simulink model "mylib2"  (R2018a)
settings: Solver=FixedStepAuto  StartTime=0.0  StopTime=10.0  RelTol=1e-3  SampleTimeConstraint=STIndependent
undefined symbols (not defined in the file or in its folder): In2, Mask_inport, Mask_outport, Out2
libraries: simulink x9
(part 2 of 2)

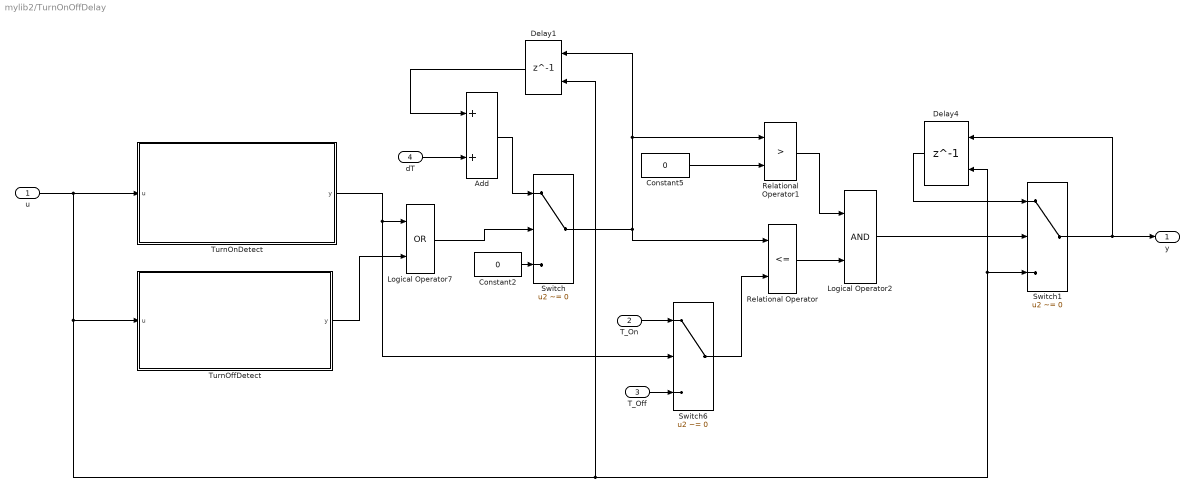
== system mylib2/TurnOnOffDelay ==
  u : Inport  OutDataTypeStr=boolean
  T_On : Inport  Port=2
  T_Off : Inport  Port=3
  dT : Inport  Port=4
  Add : Sum  RndMeth=Round  SaturateOnIntegerOverflow=on  InputSameDT=on  OutDataTypeStr=Inherit: Same as first input
  Constant2 : Constant  Value=0  OutDataTypeStr=Inherit: Inherit via back propagation
  Constant5 : Constant  Value=0  OutDataTypeStr=Inherit: Inherit via back propagation
  Delay1 : Delay  DelayLength=1  ExternalReset=Either
      settings: InputPortMap=u0,r5
  Delay4 : Delay  DelayLength=1  InitialConditionSource=Input port
      settings: InputPortMap=u0,p4
  Logical Operator2 : Logic  OutDataTypeStr=boolean
  Logical Operator7 : Logic  Operator=OR  OutDataTypeStr=boolean
  Relational Operator : RelationalOperator  Operator=<=  OutDataTypeStr=boolean  RndMeth=Simplest  InputSameDT=on
  Relational Operator1 : RelationalOperator  Operator=>  OutDataTypeStr=boolean  RndMeth=Simplest  InputSameDT=on
  Switch : Switch  Criteria=u2 ~= 0  RndMeth=Round  InputSameDT=on
  Switch1 : Switch  Criteria=u2 ~= 0
  Switch6 : Switch  Criteria=u2 ~= 0  RndMeth=Round  InputSameDT=on
  TurnOffDetect : Subsystem
  TurnOnDetect : Subsystem
  y : Outport  OutDataTypeStr=boolean
  wires:
  dT/1 -> Add/2
  Switch/1 -> Relational Operator1/1, Delay1/1, Relational Operator/1
  Delay1/1 -> Add/1
  Switch1/1 -> Delay4/1, y/1
  Add/1 -> Switch/1
  Logical Operator2/1 -> Switch1/2
  Constant2/1 -> Switch/3
  Relational Operator/1 -> Logical Operator2/2
  Relational Operator1/1 -> Logical Operator2/1
  Logical Operator7/1 -> Switch/2
  T_Off/1 -> Switch6/3
  T_On/1 -> Switch6/1
  Switch6/1 -> Relational Operator/2
  Constant5/1 -> Relational Operator1/2
  Delay4/1 -> Switch1/1
  u/1 -> Delay1/2, Delay4/2, Switch1/3, TurnOffDetect/1(u), TurnOnDetect/1(u)
  TurnOnDetect/1(y) -> Logical Operator7/1, Switch6/2
  TurnOffDetect/1(y) -> Logical Operator7/2

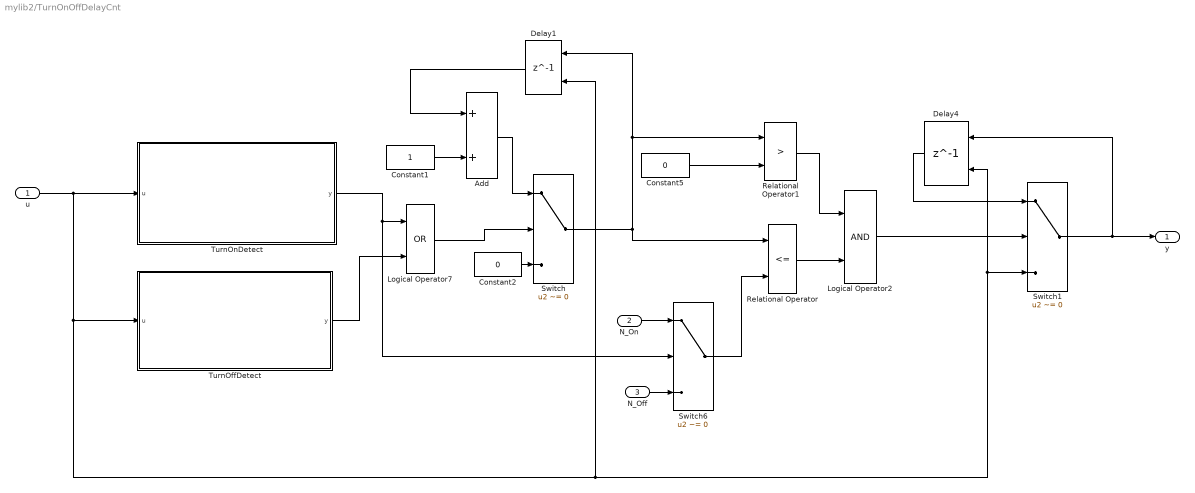
== system mylib2/TurnOnOffDelayCnt ==
  u : Inport  OutDataTypeStr=boolean
  N_On : Inport  Port=2
  N_Off : Inport  Port=3
  Add : Sum  RndMeth=Round  SaturateOnIntegerOverflow=on  InputSameDT=on  OutDataTypeStr=Inherit: Same as first input
  Constant1 : Constant  OutDataTypeStr=Inherit: Inherit via back propagation
  Constant2 : Constant  Value=0  OutDataTypeStr=Inherit: Inherit via back propagation
  Constant5 : Constant  Value=0  OutDataTypeStr=Inherit: Inherit via back propagation
  Delay1 : Delay  DelayLength=1  ExternalReset=Either
      settings: InputPortMap=u0,r5
  Delay4 : Delay  DelayLength=1  InitialConditionSource=Input port
      settings: InputPortMap=u0,p4
  Logical Operator2 : Logic  OutDataTypeStr=boolean
  Logical Operator7 : Logic  Operator=OR  OutDataTypeStr=boolean
  Relational Operator : RelationalOperator  Operator=<=  OutDataTypeStr=boolean  RndMeth=Simplest  InputSameDT=on
  Relational Operator1 : RelationalOperator  Operator=>  OutDataTypeStr=boolean  RndMeth=Simplest  InputSameDT=on
  Switch : Switch  Criteria=u2 ~= 0  RndMeth=Round  InputSameDT=on
  Switch1 : Switch  Criteria=u2 ~= 0
  Switch6 : Switch  Criteria=u2 ~= 0  RndMeth=Round  InputSameDT=on
  TurnOffDetect : Subsystem
  TurnOnDetect : Subsystem
  y : Outport  OutDataTypeStr=boolean
  wires:
  Constant1/1 -> Add/2
  Switch/1 -> Relational Operator1/1, Delay1/1, Relational Operator/1
  Delay1/1 -> Add/1
  Switch1/1 -> Delay4/1, y/1
  Add/1 -> Switch/1
  Logical Operator2/1 -> Switch1/2
  Constant2/1 -> Switch/3
  Relational Operator/1 -> Logical Operator2/2
  Relational Operator1/1 -> Logical Operator2/1
  Logical Operator7/1 -> Switch/2
  N_Off/1 -> Switch6/3
  N_On/1 -> Switch6/1
  Switch6/1 -> Relational Operator/2
  Constant5/1 -> Relational Operator1/2
  Delay4/1 -> Switch1/1
  u/1 -> Delay1/2, Delay4/2, Switch1/3, TurnOffDetect/1(u), TurnOnDetect/1(u)
  TurnOnDetect/1(y) -> Logical Operator7/1, Switch6/2
  TurnOffDetect/1(y) -> Logical Operator7/2

== system mylib2/twoAverage ==
  u1 : Inport
  u2 : Inport  Port=2
  Add : Sum  RndMeth=Round  SaturateOnIntegerOverflow=on  InputSameDT=on  OutDataTypeStr=Inherit: Same as first input
  Constant : Constant  Value=2  OutDataTypeStr=uint8
  Divide : Product  Inputs=*/  RndMeth=Round  SaturateOnIntegerOverflow=on  OutDataTypeStr=Inherit: Same as first input
  Divide1 : Product  Inputs=*/  RndMeth=Round  SaturateOnIntegerOverflow=on  OutDataTypeStr=Inherit: Same as first input
  y : Outport
  wires:
  Add/1 -> y/1
  u1/1 -> Divide/1
  Divide/1 -> Add/1
  Constant/1 -> Divide1/2, Divide/2
  u2/1 -> Divide1/1
  Divide1/1 -> Add/2

== system mylib2/F_M/Soft ==
  df : Inport  LibraryBlock=Mask_inport/In2  OutDataTypeStr=boolean
  frz : Inport  LibraryBlock=Mask_inport/In2  Port=2  OutDataTypeStr=boolean
  Delay : Delay  DelayLength=1  InitialConditionSource=Input port
      settings: InputPortMap=u0,p4
  Switch : Switch  Criteria=u2 ~= 0  InputSameDT=on
  F_M_xxx_fault_soft : Outport
  wires:
  frz/1 -> Switch/2
  Switch/1 -> Delay/1, F_M_xxx_fault_soft/1
  df/1 -> Delay/2, Switch/3
  Delay/1 -> Switch/1

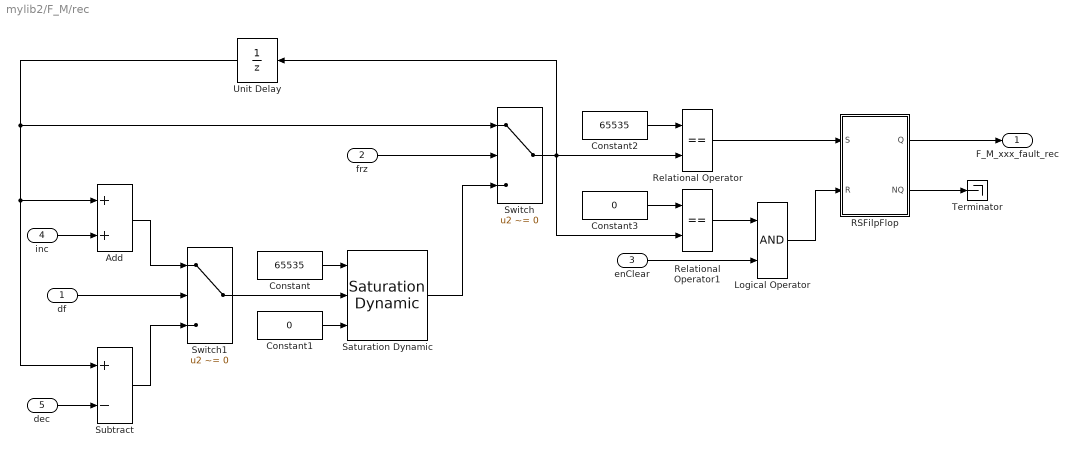
== system mylib2/F_M/rec ==
  df : Inport  LibraryBlock=Mask_inport/In2  OutDataTypeStr=boolean
  frz : Inport  LibraryBlock=Mask_inport/In2  Port=2  OutDataTypeStr=boolean
  enClear : Inport  LibraryBlock=Mask_inport/In2  Port=3  OutDataTypeStr=boolean
  inc : Inport  LibraryBlock=Mask_inport/In2  Port=4  OutDataTypeStr=uint16
  dec : Inport  LibraryBlock=Mask_inport/In2  Port=5  OutDataTypeStr=uint16
  Add : Sum  SaturateOnIntegerOverflow=on  InputSameDT=on  OutDataTypeStr=Inherit: Same as first input
  Constant : Constant  Value=65535  OutDataTypeStr=uint16
  Constant1 : Constant  Value=0  OutDataTypeStr=uint16
  Constant2 : Constant  Value=65535  OutDataTypeStr=uint16
  Constant3 : Constant  Value=0  OutDataTypeStr=uint16
  Logical Operator : Logic  AllPortsSameDT=off  OutDataTypeStr=boolean
  RSFilpFlop : Subsystem
  Relational Operator : RelationalOperator  Operator===  OutDataTypeStr=boolean  RndMeth=Simplest  InputSameDT=on
  Relational Operator1 : RelationalOperator  Operator===  OutDataTypeStr=boolean  RndMeth=Simplest  InputSameDT=on
  Saturation Dynamic : simulink/Discontinuities/Saturation Dynamic  OutMin=[]  OutMax=[]  OutDataTypeStr=Inherit: Same as second input  OutDataType=fixdt(1, 16)  OutScaling=2^-10  DoSatur=off
  Subtract : Sum  Inputs=+-  SaturateOnIntegerOverflow=on  InputSameDT=on  OutDataTypeStr=Inherit: Same as first input
  Switch : Switch  Criteria=u2 ~= 0  InputSameDT=on
  Switch1 : Switch  Criteria=u2 ~= 0  InputSameDT=on
  Terminator : Terminator
  Unit Delay : UnitDelay  SampleTime=-1
      settings: AttributesFormatString=InitialValue=%<InitialCondition>
  F_M_xxx_fault_rec : Outport  LibraryBlock=Mask_outport/Out2  OutDataTypeStr=boolean
  wires:
  df/1 -> Switch1/2
  enClear/1 -> Logical Operator/2
  dec/1 -> Subtract/2
  inc/1 -> Add/2
  frz/1 -> Switch/2
  RSFilpFlop/1(Q) -> F_M_xxx_fault_rec/1
  Unit Delay/1 -> Switch/1, Subtract/1, Add/1
  Add/1 -> Switch1/1
  Subtract/1 -> Switch1/3
  Switch1/1 -> Saturation Dynamic/2
  Constant/1 -> Saturation Dynamic/1
  Constant1/1 -> Saturation Dynamic/3
  Saturation Dynamic/1 -> Switch/3
  Constant2/1 -> Relational Operator/1
  Switch/1 -> Relational Operator1/2, Unit Delay/1, Relational Operator/2
  Constant3/1 -> Relational Operator1/1
  Relational Operator1/1 -> Logical Operator/1
  Relational Operator/1 -> RSFilpFlop/1(S)
  Logical Operator/1 -> RSFilpFlop/2(R)
  RSFilpFlop/2(NQ) -> Terminator/1

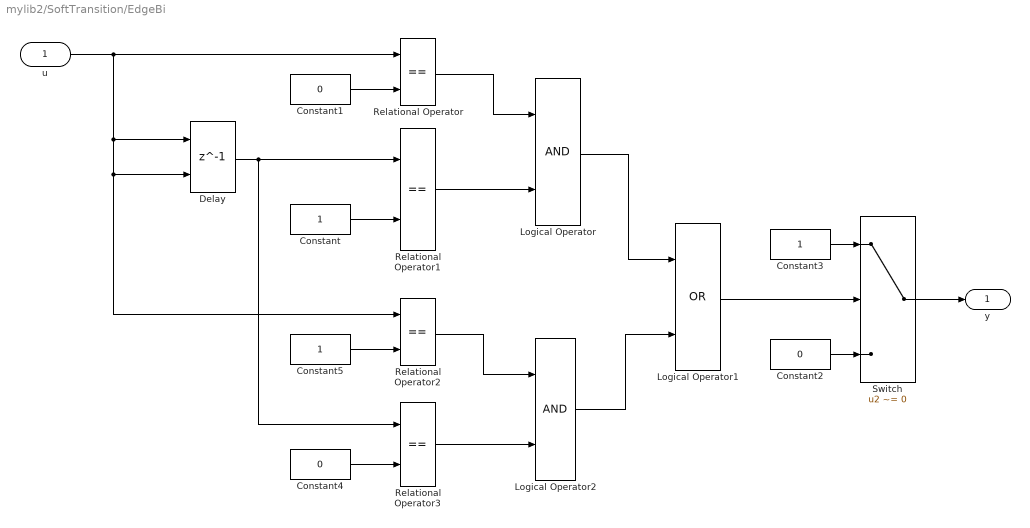
== system mylib2/SoftTransition/EdgeBi ==
  u : Inport  OutDataTypeStr=boolean
  Constant : Constant  OutDataTypeStr=boolean
  Constant1 : Constant  Value=0  OutDataTypeStr=boolean
  Constant2 : Constant  Value=0  OutDataTypeStr=boolean
  Constant3 : Constant  OutDataTypeStr=boolean
  Constant4 : Constant  Value=0  OutDataTypeStr=boolean
  Constant5 : Constant  OutDataTypeStr=boolean
  Delay : Delay  DelayLength=1  InitialConditionSource=Input port
      settings: InputPortMap=u0,p4
  Logical Operator : Logic  AllPortsSameDT=off  OutDataTypeStr=boolean
  Logical Operator1 : Logic  Operator=OR  AllPortsSameDT=off  OutDataTypeStr=boolean
  Logical Operator2 : Logic  AllPortsSameDT=off  OutDataTypeStr=boolean
  Relational Operator{,1..3} (4 alike) : RelationalOperator  Operator===  OutDataTypeStr=boolean  RndMeth=Simplest
  Switch : Switch  Criteria=u2 ~= 0
  y : Outport  OutDataTypeStr=boolean
  wires:
  Delay/1 -> Relational Operator3/1, Relational Operator1/1
  Switch/1 -> y/1
  Constant/1 -> Relational Operator1/2
  Constant1/1 -> Relational Operator/2
  Relational Operator1/1 -> Logical Operator/2
  Relational Operator/1 -> Logical Operator/1
  Constant2/1 -> Switch/3
  Constant3/1 -> Switch/1
  Logical Operator/1 -> Logical Operator1/1
  Logical Operator2/1 -> Logical Operator1/2
  u/1 -> Relational Operator2/1, Delay/2, Delay/1, Relational Operator/1
  Constant5/1 -> Relational Operator2/2
  Relational Operator2/1 -> Logical Operator2/1
  Constant4/1 -> Relational Operator3/2
  Relational Operator3/1 -> Logical Operator2/2
  Logical Operator1/1 -> Switch/2

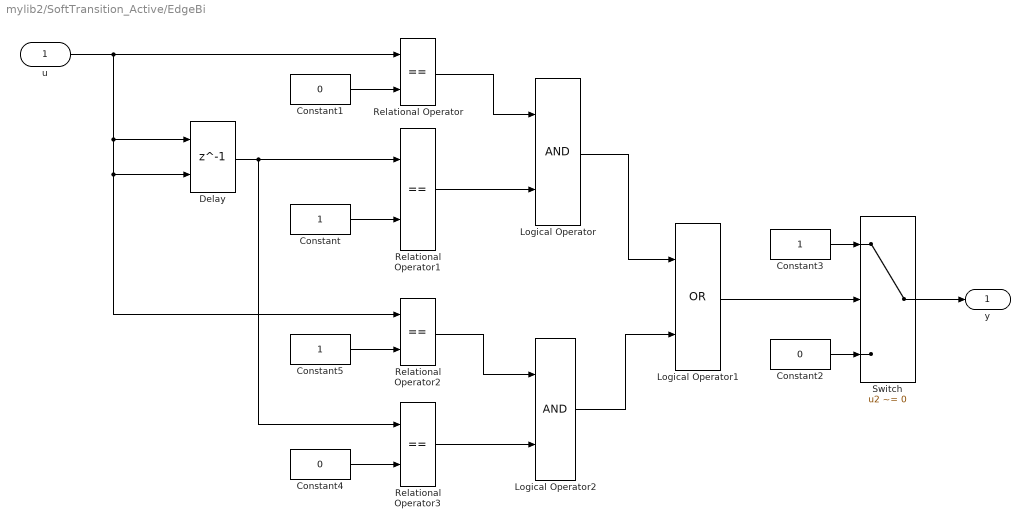
== system mylib2/SoftTransition_Active/EdgeBi ==
  u : Inport  OutDataTypeStr=boolean
  Constant : Constant  OutDataTypeStr=boolean
  Constant1 : Constant  Value=0  OutDataTypeStr=boolean
  Constant2 : Constant  Value=0  OutDataTypeStr=boolean
  Constant3 : Constant  OutDataTypeStr=boolean
  Constant4 : Constant  Value=0  OutDataTypeStr=boolean
  Constant5 : Constant  OutDataTypeStr=boolean
  Delay : Delay  DelayLength=1  InitialConditionSource=Input port
      settings: InputPortMap=u0,p4
  Logical Operator : Logic  AllPortsSameDT=off  OutDataTypeStr=boolean
  Logical Operator1 : Logic  Operator=OR  AllPortsSameDT=off  OutDataTypeStr=boolean
  Logical Operator2 : Logic  AllPortsSameDT=off  OutDataTypeStr=boolean
  Relational Operator{,1..3} (4 alike) : RelationalOperator  Operator===  OutDataTypeStr=boolean  RndMeth=Simplest
  Switch : Switch  Criteria=u2 ~= 0
  y : Outport  OutDataTypeStr=boolean
  wires:
  Delay/1 -> Relational Operator3/1, Relational Operator1/1
  Switch/1 -> y/1
  Constant/1 -> Relational Operator1/2
  Constant1/1 -> Relational Operator/2
  Relational Operator1/1 -> Logical Operator/2
  Relational Operator/1 -> Logical Operator/1
  Constant2/1 -> Switch/3
  Constant3/1 -> Switch/1
  Logical Operator/1 -> Logical Operator1/1
  Logical Operator2/1 -> Logical Operator1/2
  u/1 -> Relational Operator2/1, Delay/2, Delay/1, Relational Operator/1
  Constant5/1 -> Relational Operator2/2
  Relational Operator2/1 -> Logical Operator2/1
  Constant4/1 -> Relational Operator3/2
  Relational Operator3/1 -> Logical Operator2/2
  Logical Operator1/1 -> Switch/2

== system mylib2/SoftTransition_Rst/EdgeBi ==
  u : Inport  OutDataTypeStr=boolean
  Constant : Constant  OutDataTypeStr=boolean
  Constant1 : Constant  Value=0  OutDataTypeStr=boolean
  Constant2 : Constant  Value=0  OutDataTypeStr=boolean
  Constant3 : Constant  OutDataTypeStr=boolean
  Constant4 : Constant  Value=0  OutDataTypeStr=boolean
  Constant5 : Constant  OutDataTypeStr=boolean
  Delay : Delay  DelayLength=1  InitialConditionSource=Input port
      settings: InputPortMap=u0,p4
  Logical Operator : Logic  AllPortsSameDT=off  OutDataTypeStr=boolean
  Logical Operator1 : Logic  Operator=OR  AllPortsSameDT=off  OutDataTypeStr=boolean
  Logical Operator2 : Logic  AllPortsSameDT=off  OutDataTypeStr=boolean
  Relational Operator{,1..3} (4 alike) : RelationalOperator  Operator===  OutDataTypeStr=boolean  RndMeth=Simplest
  Switch : Switch  Criteria=u2 ~= 0
  y : Outport  OutDataTypeStr=boolean
  wires:
  Delay/1 -> Relational Operator3/1, Relational Operator1/1
  Switch/1 -> y/1
  Constant/1 -> Relational Operator1/2
  Constant1/1 -> Relational Operator/2
  Relational Operator1/1 -> Logical Operator/2
  Relational Operator/1 -> Logical Operator/1
  Constant2/1 -> Switch/3
  Constant3/1 -> Switch/1
  Logical Operator/1 -> Logical Operator1/1
  Logical Operator2/1 -> Logical Operator1/2
  u/1 -> Relational Operator2/1, Delay/2, Delay/1, Relational Operator/1
  Constant5/1 -> Relational Operator2/2
  Relational Operator2/1 -> Logical Operator2/1
  Constant4/1 -> Relational Operator3/2
  Relational Operator3/1 -> Logical Operator2/2
  Logical Operator1/1 -> Switch/2

== system mylib2/TimerDwn/EdgeRising ==
  u : Inport  OutDataTypeStr=boolean
  Constant : Constant  Value=0  OutDataTypeStr=boolean
  Constant1 : Constant  OutDataTypeStr=boolean
  Constant2 : Constant  Value=0  OutDataTypeStr=boolean
  Constant3 : Constant  OutDataTypeStr=boolean
  Delay : Delay  DelayLength=1  InitialConditionSource=Input port
      settings: InputPortMap=u0,p4
  Logical Operator : Logic  AllPortsSameDT=off  OutDataTypeStr=boolean
  Relational Operator : RelationalOperator  Operator===  OutDataTypeStr=boolean  RndMeth=Simplest
  Relational Operator1 : RelationalOperator  Operator===  OutDataTypeStr=boolean  RndMeth=Simplest
  Switch : Switch  Criteria=u2 ~= 0
  y : Outport  OutDataTypeStr=boolean
  wires:
  Logical Operator/1 -> Switch/2
  Switch/1 -> y/1
  u/1 -> Delay/1, Delay/2, Relational Operator/1
  Constant1/1 -> Relational Operator/2
  Constant/1 -> Relational Operator1/2
  Delay/1 -> Relational Operator1/1
  Relational Operator/1 -> Logical Operator/1
  Relational Operator1/1 -> Logical Operator/2
  Constant2/1 -> Switch/3
  Constant3/1 -> Switch/1

== system mylib2/TurnOnOffDelay/TurnOffDetect ==
  u : Inport
  Constant6 : Constant  OutDataTypeStr=boolean
  Constant7 : Constant  Value=0  OutDataTypeStr=boolean
  Constant9 : Constant  OutDataTypeStr=boolean
  Delay3 : Delay  DelayLength=1  InitialConditionSource=Input port
      settings: InputPortMap=u0,p4
  Delay5 : Delay  DelayLength=1  ExternalReset=Rising
      settings: InputPortMap=u0,r5
  Equal2 : RelationalOperator  Operator===  OutDataTypeStr=boolean  RndMeth=Simplest  InputSameDT=on
  Equal3 : RelationalOperator  Operator===  OutDataTypeStr=boolean  RndMeth=Simplest  InputSameDT=on
  Logical Operator3 : Logic  OutDataTypeStr=boolean
  Logical Operator4 : Logic  OutDataTypeStr=boolean
  Logical Operator6 : Logic  Operator=NOT  AllPortsSameDT=off  OutDataTypeStr=boolean
  Switch5 : Switch  Criteria=u2 ~= 0  RndMeth=Round  InputSameDT=on
  y : Outport
  wires:
  Equal3/1 -> Logical Operator3/2
  Logical Operator6/1 -> Logical Operator4/2
  Constant7/1 -> Equal3/2
  Switch5/1 -> Delay5/1, Logical Operator4/1
  Equal2/1 -> Logical Operator3/1
  Delay5/1 -> Switch5/3
  Constant6/1 -> Equal2/2
  Constant9/1 -> Switch5/1
  Logical Operator3/1 -> Switch5/2
  Delay3/1 -> Equal2/1
  u/1 -> Logical Operator6/1, Delay5/2, Equal3/1, Delay3/2, Delay3/1
  Logical Operator4/1 -> y/1

== system mylib2/TurnOnOffDelay/TurnOnDetect ==
  u : Inport  OutDataTypeStr=boolean
  Constant : Constant  Value=0  OutDataTypeStr=boolean
  Constant1 : Constant  OutDataTypeStr=boolean
  Constant3 : Constant  OutDataTypeStr=boolean
  Delay : Delay  DelayLength=1  InitialConditionSource=Input port
      settings: InputPortMap=u0,p4
  Delay2 : Delay  DelayLength=1  ExternalReset=Falling
      settings: InputPortMap=u0,r5
  Equal : RelationalOperator  Operator===  OutDataTypeStr=boolean  RndMeth=Simplest  InputSameDT=on
  Equal1 : RelationalOperator  Operator===  OutDataTypeStr=boolean  RndMeth=Simplest  InputSameDT=on
  Logical Operator : Logic  OutDataTypeStr=boolean
  Logical Operator1 : Logic  OutDataTypeStr=boolean
  Switch2 : Switch  Criteria=u2 ~= 0  RndMeth=Round  InputSameDT=on
  y : Outport
  wires:
  Constant3/1 -> Switch2/1
  Constant/1 -> Equal/2
  Switch2/1 -> Delay2/1, Logical Operator1/1
  Equal1/1 -> Logical Operator/2
  Logical Operator1/1 -> y/1
  Equal/1 -> Logical Operator/1
  Delay/1 -> Equal/1
  Delay2/1 -> Switch2/3
  Logical Operator/1 -> Switch2/2
  Constant1/1 -> Equal1/2
  u/1 -> Delay/2, Logical Operator1/2, Delay2/2, Equal1/1, Delay/1

== system mylib2/TurnOnOffDelayCnt/TurnOffDetect ==
  u : Inport
  Constant6 : Constant  OutDataTypeStr=boolean
  Constant7 : Constant  Value=0  OutDataTypeStr=boolean
  Constant9 : Constant  OutDataTypeStr=boolean
  Delay3 : Delay  DelayLength=1  InitialConditionSource=Input port
      settings: InputPortMap=u0,p4
  Delay5 : Delay  DelayLength=1  ExternalReset=Rising
      settings: InputPortMap=u0,r5
  Equal2 : RelationalOperator  Operator===  OutDataTypeStr=boolean  RndMeth=Simplest  InputSameDT=on
  Equal3 : RelationalOperator  Operator===  OutDataTypeStr=boolean  RndMeth=Simplest  InputSameDT=on
  Logical Operator3 : Logic  OutDataTypeStr=boolean
  Logical Operator4 : Logic  OutDataTypeStr=boolean
  Logical Operator6 : Logic  Operator=NOT  AllPortsSameDT=off  OutDataTypeStr=boolean
  Switch5 : Switch  Criteria=u2 ~= 0  RndMeth=Round  InputSameDT=on
  y : Outport
  wires:
  Equal3/1 -> Logical Operator3/2
  Logical Operator6/1 -> Logical Operator4/2
  Constant7/1 -> Equal3/2
  Switch5/1 -> Delay5/1, Logical Operator4/1
  Equal2/1 -> Logical Operator3/1
  Delay5/1 -> Switch5/3
  Constant6/1 -> Equal2/2
  Constant9/1 -> Switch5/1
  Logical Operator3/1 -> Switch5/2
  Delay3/1 -> Equal2/1
  u/1 -> Logical Operator6/1, Delay5/2, Equal3/1, Delay3/2, Delay3/1
  Logical Operator4/1 -> y/1

== system mylib2/TurnOnOffDelayCnt/TurnOnDetect ==
  u : Inport  OutDataTypeStr=boolean
  Constant : Constant  Value=0  OutDataTypeStr=boolean
  Constant1 : Constant  OutDataTypeStr=boolean
  Constant3 : Constant  OutDataTypeStr=boolean
  Delay : Delay  DelayLength=1  InitialConditionSource=Input port
      settings: InputPortMap=u0,p4
  Delay2 : Delay  DelayLength=1  ExternalReset=Falling
      settings: InputPortMap=u0,r5
  Equal : RelationalOperator  Operator===  OutDataTypeStr=boolean  RndMeth=Simplest  InputSameDT=on
  Equal1 : RelationalOperator  Operator===  OutDataTypeStr=boolean  RndMeth=Simplest  InputSameDT=on
  Logical Operator : Logic  OutDataTypeStr=boolean
  Logical Operator1 : Logic  OutDataTypeStr=boolean
  Switch2 : Switch  Criteria=u2 ~= 0  RndMeth=Round  InputSameDT=on
  y : Outport
  wires:
  Constant3/1 -> Switch2/1
  Constant/1 -> Equal/2
  Switch2/1 -> Delay2/1, Logical Operator1/1
  Equal1/1 -> Logical Operator/2
  Logical Operator1/1 -> y/1
  Equal/1 -> Logical Operator/1
  Delay/1 -> Equal/1
  Delay2/1 -> Switch2/3
  Logical Operator/1 -> Switch2/2
  Constant1/1 -> Equal1/2
  u/1 -> Delay/2, Logical Operator1/2, Delay2/2, Equal1/1, Delay/1

== system mylib2/F_M/rec/RSFilpFlop ==
  note: S
      | R
      | Q
      | NQ
      |
      | 0
      | 1
      | 0
      | 1
      |
      | 1
      | 0
      | 1
      | 0
      |
      | 0
      | 0
      | Qn-1
      | !Qn-1
      |
      | 1
      | 1
      | 0
      | 0
  S : Inport  OutDataTypeStr=boolean
  R : Inport  Port=2  OutDataTypeStr=boolean
  Constant : Constant  Value=0  OutDataTypeStr=boolean
  Constant1 : Constant  OutDataTypeStr=boolean
  Constant2 : Constant  Value=0  OutDataTypeStr=boolean
  Constant3 : Constant  OutDataTypeStr=boolean
  Logical Operator : Logic  Operator=NOT  AllPortsSameDT=off  OutDataTypeStr=boolean
  Switch{,1..3} (4 alike) : Switch  Criteria=u2 ~= 0
  Unit Delay : UnitDelay  SampleTime=-1
      settings: AttributesFormatString=InitialValue=%<InitialCondition>
  Q : Outport  OutDataTypeStr=boolean
  NQ : Outport  Port=2  OutDataTypeStr=boolean
  wires:
  R/1 -> Switch3/2, Switch/2
  Constant/1 -> Switch/1
  Switch/1 -> Unit Delay/1, Q/1
  S/1 -> Switch2/2, Switch1/2
  Constant1/1 -> Switch1/1
  Switch1/1 -> Switch/3
  Unit Delay/1 -> Switch1/3, Logical Operator/1
  Switch2/1 -> NQ/1
  Constant2/1 -> Switch2/1
  Switch3/1 -> Switch2/3
  Constant3/1 -> Switch3/1
  Logical Operator/1 -> Switch3/3
